simulink model "test_sensor_plc_actuator"  (R2014a)
settings: Solver=ode45  StartTime=0.0  StopTime=10  RelTol=1e-3
libraries: TEsim_utils x5
settings Model: Creator=rnc4  LastModifiedBy=rnc4

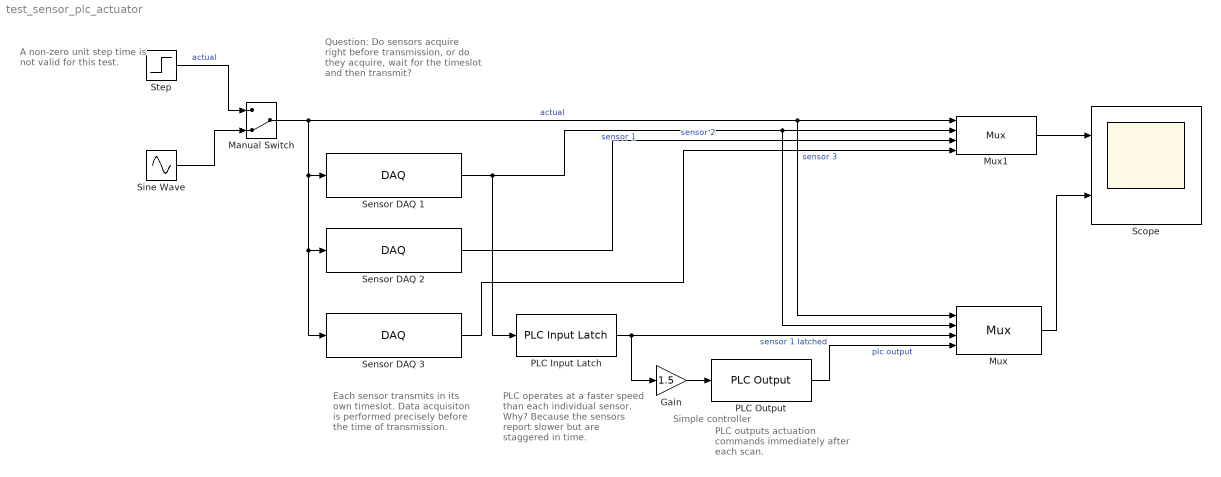
== system test_sensor_plc_actuator ==
  note: PLC outputs actuation commands immediately after each scan.
  note: Simple controller
  note: PLC operates at a faster speed than each individual sensor. Why? Because the sensors report slower but are staggered in time.
  note: A non-zero unit step time is not valid for this test.
  note: Each sensor transmits in its own timeslot. Data acquisiton is performed precisely before the time of transmission.
  note: Question: Do sensors acquire right before transmission, or do they acquire, wait for the timeslot and then transmit?
  Gain : Gain  Gain=1.5
  Manual Switch : ManualSwitch  CurrentSetting=0
  Mux : Mux
      settings: DisplayOption=signals
  Mux1 : Mux
      settings: DisplayOption=signals
  PLC Input Latch : TEsim_utils/PLC Input Latch  polling_time_sec=0.1  polling_offset_sec=0
  PLC Output : TEsim_utils/PLC Output
  Scope : Scope  NumInputPorts=2
      settings: ShowLegends=on  TimeRange=10  YMin=-6~-8  YMax=6~8
  Sensor DAQ 1 : TEsim_utils/DAQ  frame_dur_sec=1  timeslot_offset_ms=0
  Sensor DAQ 2 : TEsim_utils/DAQ  frame_dur_sec=1  timeslot_offset_ms=20
  Sensor DAQ 3 : TEsim_utils/DAQ  frame_dur_sec=1  timeslot_offset_ms=80
  Sine Wave : Sin  Amplitude=5  Frequency=0.25*pi  SampleTime=1/1000
  Step : Step  Time=0  SampleTime=1/1000
  wires:
  Manual Switch/1 -> Mux/1, Mux1/1, Sensor DAQ 1/1, Sensor DAQ 3/1, Sensor DAQ 2/1  "actual"
  Sine Wave/1 -> Manual Switch/2
  Step/1 -> Manual Switch/1  "actual"
  Gain/1 -> PLC Output/1
  Mux/1 -> Scope/2
  PLC Output/1 -> Mux/4  "plc output"
  Mux1/1 -> Scope/1
  Sensor DAQ 2/1 -> Mux1/3  "sensor 2"
  Sensor DAQ 3/1 -> Mux1/4  "sensor 3"
  Sensor DAQ 1/1 -> PLC Input Latch/1, Mux/2, Mux1/2  "sensor 1"
  PLC Input Latch/1 -> Mux/3, Gain/1  "sensor 1 latched"
